simulink model "flex_robot_flat"  (R2020b)
settings: Solver=ode45  StartTime=0.0  StopTime=40  RelTol=1e-3
InitFcn:
  | params;
values from neighbouring files (symbols this model uses):
  param_controller = [c,d__1,d__2,m,g,l,I__1,I__2]    [params.m]
  param_system = [c,d__1,d__2,m,g,l,I__1,I__2]    [params.m]
  param_system_altered1 = [c*1.1,d__1,d__2,m,g,l,I__1,I__2]    [params.m]
  param_system_altered2 = [c*0.6,d__1,d__2,m,g,l,I__1,I__2]    [params.m]
  x__0 = [-pi/2,-pi/2,0,0]    [params.m]
undefined symbols (not defined in the file or in its folder): parReg
libraries: simulink_extras x6
settings Model: Creator=me  LastModifiedBy=simon
settings DataIOCC: LimitDataPoints=on  SaveFormat=Array  ReturnWorkspaceOutputs=off
settings OptimizationCC: BlockReduction=off  BooleanDataType=off  LifeSpan=inf
settings DebuggingCC: SaveWithParameterizedLinksMsg=none  UnderspecifiedInitializationDetection=Classic  MergeDetectMultiDrivingBlocksExec=none  SignalResolutionControl=TryResolveAllWithWarning  SFUnexpectedBacktrackingDiag=warning  SFNoUnconditionalDefaultTransitionDiag=warning  SFExecutionAtInitializationDiag=none  ArithmeticOperatorsInVariantConditions=warning
settings HardwareCC: ProdBitPerPointer=32  ProdBitPerSizeT=32  ProdBitPerPtrDiffT=32  ProdLargestAtomicFloat=None  ProdIntDivRoundTo=Undefined  ProdEndianess=Unspecified  ProdWordSize=32  ProdHWDeviceType=32-bit Generic  TargetUnknown=on
settings ModelReferenceCC: PropagateSignalLabelsOutOfModel=off
settings SFSimCC: SimUseLocalCustomCode=off  CustomCodeUndefinedFunction=UseInterfaceOnly
settings RTWCC: RTWUseLocalCustomCode=off
settings CodeAppCC: StateflowObjectComments=on
settings GRTTargetCC: TargetLangStandard=C89/C90 (ANSI)
settings ConfigComp: CovMetricSettings=dw  CovSaveCumulativeToWorkspaceVar=on  CovSaveSingleToWorkspaceVar=on  CovExternalEMLEnable=off

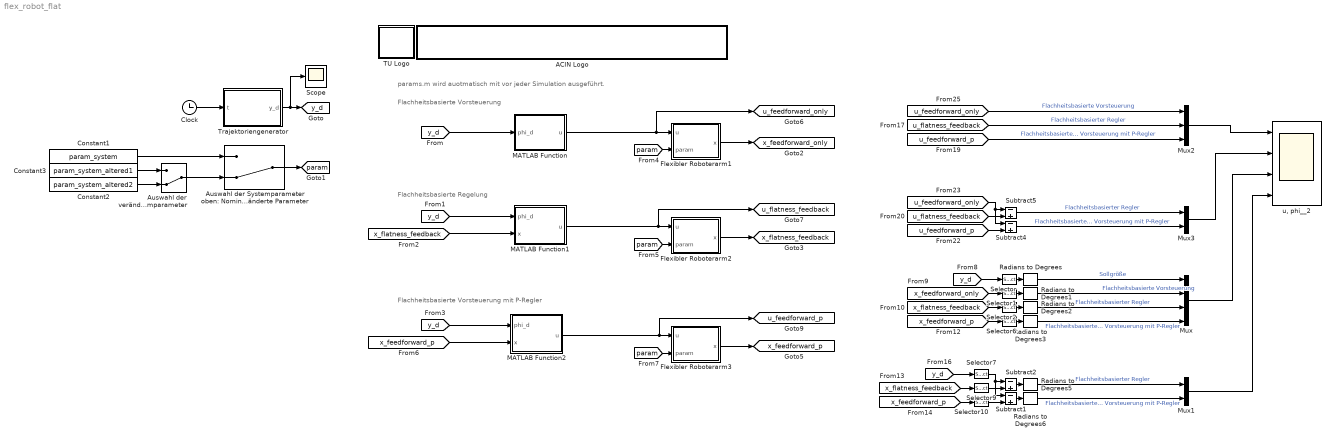
== system flex_robot_flat ==
  note: Flachheitsbasierte Vorsteuerung
  note: Flachheitsbasierte Regelung
  note: Flachheitsbasierte Vorsteuerung mit P-Regler
  note: params.m wird auotmatisch mit vor jeder Simulation ausgeführt.
  ACIN Logo : Subsystem
      mask init:
      | s = get_param(gcb,'UserData');
      mask Display:
      | image(s.logo,[0 0 439 45]);
      | %axis image
  Auswahl der veränderten Systemparameter : ManualSwitch  CurrentSetting=0
  Auswahl der Systemparameter oben: Nominelle Parameter unten: Veränderte Parameter : ManualSwitch  CurrentSetting=0
  Clock : Clock
  Constant1 : Constant  Value=param_system
  Constant2 : Constant  Value=param_system_altered2
  Constant3 : Constant  Value=param_system_altered1
  Flexibler Roboterarm1 : Subsystem
  Flexibler Roboterarm2 : Subsystem
  Flexibler Roboterarm3 : Subsystem
  MATLAB Function : MATLAB Function  TreatAsAtomicUnit=on
  MATLAB Function1 : MATLAB Function  TreatAsAtomicUnit=on
  MATLAB Function2 : MATLAB Function  TreatAsAtomicUnit=on
  Mux : Mux
  Mux1 : Mux  Inputs=2
  Mux2 : Mux  Inputs=3
  Mux3 : Mux  Inputs=2
  Radians to Degrees{,1..3,5..6} (6 alike) : simulink_extras/Transformations/Radians to Degrees
  Scope : Scope
  Selector : Selector  InputPortWidth=5  IndexOptions=Index vector (dialog)  Indices=[1]  OutputSizes=1
  Selector{1..2,6,9..10} (5 alike) : Selector  InputPortWidth=4  IndexOptions=Index vector (dialog)  Indices=2  OutputSizes=1
  Selector7 : Selector  InputPortWidth=5  IndexOptions=Index vector (dialog)  Indices=[1]  OutputSizes=1
  Subtract{1..2,4..5} (4 alike) : Sum  Inputs=-+
  TU Logo : Subsystem
      mask init:
      | s = get_param(gcb,'UserData');
      mask Display: image(s.logo,[0 0 45 45]);
  Trajektoriengenerator : MATLAB Function  TreatAsAtomicUnit=on
  "u, phi__2" : Scope  NumInputPorts=4
  tag scope: param=global, u_feedforward_only=global, u_feedforward_p=global, u_flatness_feedback=global, x_feedforward_only=global, x_feedforward_p=global, x_flatness_feedback=global, y_d=global
  wires:
  Clock/1 -> Trajektoriengenerator/1(t)
  Radians to Degrees/1 -> Mux/1  "Sollgröße"
  MATLAB Function1/1(u) -> [u_flatness_feedback], Flexibler Roboterarm2/1(u)
  Flexibler Roboterarm2/1(x) -> [x_flatness_feedback]
  Flexibler Roboterarm3/1(x) -> [x_feedforward_p]
  MATLAB Function2/1(u) -> [u_feedforward_p], Flexibler Roboterarm3/1(u)
  Constant1/1 -> Auswahl der Systemparameter oben: Nominelle Parameter unten: Veränderte Parameter/1
  Trajektoriengenerator/1(y_d) -> Scope/1, [y_d]
  [y_d] -> MATLAB Function/1(phi_d)
  [y_d] -> MATLAB Function1/1(phi_d)
  [y_d] -> MATLAB Function2/1(phi_d)
  Auswahl der Systemparameter oben: Nominelle Parameter unten: Veränderte Parameter/1 -> [param]
  [param] -> Flexibler Roboterarm1/2(param)
  [param] -> Flexibler Roboterarm2/2(param)
  [param] -> Flexibler Roboterarm3/2(param)
  Flexibler Roboterarm1/1(x) -> [x_feedforward_only]
  [y_d] -> Selector/1
  [x_feedforward_only] -> Selector1/1
  Radians to Degrees1/1 -> Mux/2  "Flachheitsbasierte Vorsteuerung"
  Radians to Degrees2/1 -> Mux/3  "Flachheitsbasierter Regler"
  [x_flatness_feedback] -> Selector2/1
  Radians to Degrees5/1 -> Mux1/1  "Flachheitsbasierter Regler"
  [x_feedforward_p] -> Selector10/1
  [x_flatness_feedback] -> Selector9/1
  Radians to Degrees6/1 -> Mux1/2  "Flachheitsbasierte Vorsteuerung mit P-Regler"
  Selector9/1 -> Subtract2/2
  Selector10/1 -> Subtract1/2
  Selector7/1 -> Subtract1/1, Subtract2/1
  [u_flatness_feedback] -> Mux2/2  "Flachheitsbasierter Regler"
  Subtract4/1 -> Mux3/2  "Flachheitsbasierte Vorsteuerung mit P-Regler"
  [u_flatness_feedback] -> Subtract5/2
  [u_feedforward_only] -> Subtract4/1, Subtract5/1
  Mux2/1 -> "u, phi__2"/1
  [u_feedforward_p] -> Subtract4/2
  Subtract5/1 -> Mux3/1  "Flachheitsbasierter Regler"
  [u_feedforward_only] -> Mux2/1  "Flachheitsbasierte Vorsteuerung"
  Mux3/1 -> "u, phi__2"/2
  Constant3/1 -> Auswahl der veränderten Systemparameter/1
  Constant2/1 -> Auswahl der veränderten Systemparameter/2
  Auswahl der veränderten Systemparameter/1 -> Auswahl der Systemparameter oben: Nominelle Parameter unten: Veränderte Parameter/2
  Radians to Degrees3/1 -> Mux/4  "Flachheitsbasierte Vorsteuerung mit P-Regler"
  [x_feedforward_p] -> Selector6/1
  [y_d] -> Selector7/1
  [u_feedforward_p] -> Mux2/3  "Flachheitsbasierte Vorsteuerung mit P-Regler"
  MATLAB Function/1(u) -> [u_feedforward_only], Flexibler Roboterarm1/1(u)
  Mux/1 -> "u, phi__2"/3
  Mux1/1 -> "u, phi__2"/4
  Selector/1 -> Radians to Degrees/1
  Selector1/1 -> Radians to Degrees1/1
  Selector2/1 -> Radians to Degrees2/1
  Selector6/1 -> Radians to Degrees3/1
  Subtract2/1 -> Radians to Degrees5/1
  Subtract1/1 -> Radians to Degrees6/1
  [x_flatness_feedback] -> MATLAB Function1/2(x)
  [x_feedforward_p] -> MATLAB Function2/2(x)

== system flex_robot_flat/ACIN Logo ==

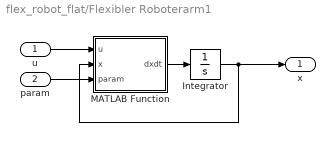
== system flex_robot_flat/Flexibler Roboterarm1 ==
  u : Inport
  param : Inport  Port=2
  Integrator : Integrator  InitialCondition=x__0
  MATLAB Function : MATLAB Function  TreatAsAtomicUnit=on
  x : Outport  VectorParamsAs1DForOutWhenUnconnected=off
  wires:
  u/1 -> MATLAB Function/1(u)
  Integrator/1 -> x/1, MATLAB Function/2(x)
  MATLAB Function/1(dxdt) -> Integrator/1
  param/1 -> MATLAB Function/3(param)

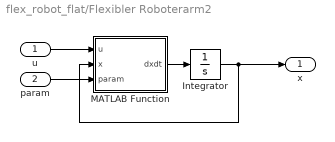
== system flex_robot_flat/Flexibler Roboterarm2 ==
  u : Inport
  param : Inport  Port=2
  Integrator : Integrator  InitialCondition=x__0
  MATLAB Function : MATLAB Function  TreatAsAtomicUnit=on
  x : Outport  VectorParamsAs1DForOutWhenUnconnected=off
  wires:
  u/1 -> MATLAB Function/1(u)
  Integrator/1 -> x/1, MATLAB Function/2(x)
  MATLAB Function/1(dxdt) -> Integrator/1
  param/1 -> MATLAB Function/3(param)

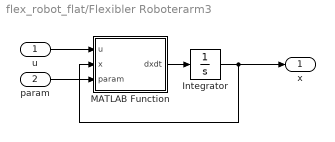
== system flex_robot_flat/Flexibler Roboterarm3 ==
  u : Inport
  param : Inport  Port=2
  Integrator : Integrator  InitialCondition=x__0
  MATLAB Function : MATLAB Function  TreatAsAtomicUnit=on
  x : Outport  VectorParamsAs1DForOutWhenUnconnected=off
  wires:
  u/1 -> MATLAB Function/1(u)
  Integrator/1 -> x/1, MATLAB Function/2(x)
  MATLAB Function/1(dxdt) -> Integrator/1
  param/1 -> MATLAB Function/3(param)

== system flex_robot_flat/TU Logo ==

== matlab function flex_robot_flat/MATLAB Function1 ==
  data: phi_d input; x input; u output; param_controller parameter; parReg parameter
function u = fcn(phi_d,x,param_controller,parReg)

% Sollwerte von phi2 und dessen Ableitungen
z__1 = phi_d(1);
z__2 = phi_d(2);
z__3 = phi_d(3);
z__4 = phi_d(4);
dz__4 = phi_d(5);

% Parameter des Systems
c = param_controller(1);
d__1 = param_controller(2);
d__2 = param_controller(3);
m = param_controller(4);
g = param_controller(5);
l = param_controller(6);
I__1 = param_controller(7);
I__2 = param_controller(8);

% Messgrößen
varphi__1 = x(1);
varphi__2 = x(2);
omega__1 = x(3);
omega__2 = x(4);

% Reglerparameter
a0 = parReg.a0;
a1 = parReg.a1;
a2 = parReg.a2;
a3 = parReg.a3;

% Stellgröße
u = 0.1e1 / c * I__2 * I__1 * (dz__4 + d__2 / I__2 ^ 2 * c * omega__1 - (m * g * l * cos(varphi__2) / I__2 * omega__2 - d__2 / I__2 ^ 2 * (-c + m * g * l * sin(varphi__2))) * omega__2 - c / I__2 * (-c * varphi__1 + c * varphi__2 - d__1 * omega__1) / I__1 - ((-c + m * g * l * sin(varphi__2)) / I__2 + d__2 ^ 2 / I__2 ^ 2) * (c * varphi__1 - c * varphi__2 - m * g * l * cos(varphi__2) - d__2 * omega__2) / I__2 - a0 * (-z__1 + varphi__2) - a1 * (-z__2 + omega__2) - a2 * ((c * varphi__1 - c * varphi__2 - m * g * l * cos(varphi__2) - d__2 * omega__2) / I__2 - z__3) - a3 * (c / I__2 * omega__1 + (-c + m * g * l * sin(varphi__2)) / I__2 * omega__2 - d__2 / I__2 ^ 2 * (c * varphi__1 - c * varphi__2 - m * g * l * cos(varphi__2) - d__2 * omega__2) - z__4));

== matlab function flex_robot_flat/MATLAB Function ==
  data: phi_d input; u output; param_controller parameter
function u = fcn(phi_d,param_controller)

% Sollwerte von phi2 und dessen Ableitungen
z__1 = phi_d(1);
z__2 = phi_d(2);
z__3 = phi_d(3);
z__4 = phi_d(4);
dz__4 = phi_d(5);

% Parameter des Systems
c = param_controller(1);
d__1 = param_controller(2);
d__2 = param_controller(3);
m = param_controller(4);
g = param_controller(5);
l = param_controller(6);
I__1 = param_controller(7);
I__2 = param_controller(8);

varphi__1 = (m * g * l * cos(z__1) + z__3 * I__2 + c * z__1 + d__2 * z__2) / c;
varphi__2 = z__1;
omega__1 = (-sin(z__1) * g * l * m * z__2 + I__2 * z__4 + c * z__2 + d__2 * z__3) / c;
omega__2 = z__2;

% Stellgröße
u = 0.1e1 / c * I__2 * I__1 * (d__2 / I__2 ^ 2 * c * omega__1 - (m * g * l * cos(varphi__2) / I__2 * omega__2 - d__2 / I__2 ^ 2 * (-c + m * g * l * sin(varphi__2))) * omega__2 - c / I__2 * (-c * varphi__1 + c * varphi__2 - d__1 * omega__1) / I__1 - ((-c + m * g * l * sin(varphi__2)) / I__2 + d__2 ^ 2 / I__2 ^ 2) * (c * varphi__1 - c * varphi__2 - m * g * l * cos(varphi__2) - d__2 * omega__2) / I__2 + dz__4);

== matlab function flex_robot_flat/MATLAB Function2 ==
  data: phi_d input; x input; u output; param_controller parameter; parReg parameter
function u = fcn(phi_d,x,param_controller,parReg)

% Sollwerte von phi2 und dessen Ableitungen
z__1 = phi_d(1);
z__2 = phi_d(2);
z__3 = phi_d(3);
z__4 = phi_d(4);
dz__4 = phi_d(5);

% Parameter des Systems
c = param_controller(1);
d__1 = param_controller(2);
d__2 = param_controller(3);
m = param_controller(4);
g = param_controller(5);
l = param_controller(6);
I__1 = param_controller(7);
I__2 = param_controller(8);

varphi__1 = (m * g * l * cos(z__1) + z__3 * I__2 + c * z__1 + d__2 * z__2) / c;
varphi__2 = z__1;
omega__1 = (-sin(z__1) * g * l * m * z__2 + I__2 * z__4 + c * z__2 + d__2 * z__3) / c;
omega__2 = z__2;

% Fehler
e = z__1-x(2);

% Stellgröße
u = 0.1e1 / c * I__2 * I__1 * (d__2 / I__2 ^ 2 * c * omega__1 - (m * g * l * cos(varphi__2) / I__2 * omega__2 - d__2 / I__2 ^ 2 * (-c + m * g * l * sin(varphi__2))) * omega__2 - c / I__2 * (-c * varphi__1 + c * varphi__2 - d__1 * omega__1) / I__1 - ((-c + m * g * l * sin(varphi__2)) / I__2 + d__2 ^ 2 / I__2 ^ 2) * (c * varphi__1 - c * varphi__2 - m * g * l * cos(varphi__2) - d__2 * omega__2) / I__2 + dz__4);
u = u + parReg.K*e;

== matlab function flex_robot_flat/Trajektoriengenerator ==
  data: t input; y_d output; param_trajectory parameter
function y_d  = trajgen(t,param_trajectory)
  T   = param_trajectory(1);
  a0 = param_trajectory(2);
  a1 = param_trajectory(3);

  % Generierung der Trajektorie y1d für den flachen Ausgang y1
  if (t<=0)
      phi__2_d     = a0;
      phi__2_dp    = 0;
      phi__2_dpp   = 0;
      phi__2_dppp  = 0;
      phi__2_dpppp = 0;
  elseif (t>T)
      phi__2_d     = a1;
      phi__2_dp    = 0;
      phi__2_dpp   = 0;
      phi__2_dppp  = 0;
      phi__2_dpppp = 0;
  else
      % Generierung der Solltrajektorie für q1
      phi__2_d     = a0 - 126 / T ^ 5 * (a0 - a1) * t ^ 5 + 420 / T ^ 6 * (a0 ...
          - a1) * t ^ 6 - 540 / T ^ 7 * (a0 - a1) * t ^ 7 + 315 / T ^ 8 * ...
          (a0 - a1) * t ^ 8 - 70 * (a0 - a1) / T ^ 9 * t ^ 9;
      % Generierung der ersten Ableitung der Solltrajektorie für q1
      phi__2_dp    = -630 / T ^ 5 * (a0 - a1) * t ^ 4 + 2520 / T ^ 6 * (a0 - ...
          a1) * t ^ 5 - 3780 / T ^ 7 * (a0 - a1) * t ^ 6 + 2520 / T ^ 8 * ...
          (a0 - a1) * t ^ 7 - 630 * (a0 - a1) / T ^ 9 * t ^ 8;
      % Generierung der zweiten Ableitung der Solltrajektorie für q1
      phi__2_dpp   =  -2520 / T ^ 5 * (a0 - a1) * t ^ 3 + 12600 / T ^ 6 * (a0 - ...
          a1) * t ^ 4 - 22680 / T ^ 7 * (a0 - a1) * t ^ 5 + 17640 / T ^ 8 * ...
          (a0 - a1) * t ^ 6 - 5040 * (a0 - a1) / T ^ 9 * t ^ 7;
      % Generierung der dritten Ableitung der Solltrajektorie für q1
      phi__2_dppp  = -7560 / T ^ 5 * (a0 - a1) * t ^ 2 + 50400 / T ^ 6 * (a0 - ...
          a1) * t ^ 3 - 113400 / T ^ 7 * (a0 - a1) * t ^ 4 + 105840 / T ^ 8 ...
          * (a0 - a1) * t ^ 5 - 35280 * (a0 - a1) / T ^ 9 * t ^ 6;
      % Generierung der vierten Ableitung der Solltrajektorie für q1
      phi__2_dpppp =  -15120 / T ^ 5 * (a0 - a1) * t + 151200 / T ^ 6 * (a0 - ...
          a1) * t ^ 2 - 453600 / T ^ 7 * (a0 - a1) * t ^ 3 + 529200 / T ^ 8 ...
          * (a0 - a1) * t ^ 4 - 211680 * (a0 - a1) / T ^ 9 * t ^ 5;
  end
  % Verpacken der Solltrajektorie samt Ableitungen in einem Vektor zur Uebergabe
  % an die Vorsteuerung
  y_d = [phi__2_d,phi__2_dp,phi__2_dpp,phi__2_dppp,phi__2_dpppp];
end

== matlab function flex_robot_flat/Flexibler Roboterarm2/MATLAB Function ==
  data: u input; dxdt output; x input; param input
function dxdt = fcn(u,x,param)
  c=param(1);
  d__1=param(2);
  d__2=param(3);
  m=param(4);
  g=param(5);
  l=param(6);
  I__1=param(7);
  I__2=param(8);
  
  varphi__1=x(1);
  varphi__2=x(2);
  omega__1=x(3);
  omega__2=x(4);
  
  dxdt=zeros(4,1);
  dxdt(1) = omega__1;
  dxdt(2) = omega__2;
  dxdt(3) = -c/I__1*varphi__1 + c/I__1*varphi__2 - d__1/I__1*omega__1 + 1/I__1*u;
  dxdt(4) =  c/I__2*varphi__1 - c/I__2*varphi__2 - m*g*l/I__2*cos(varphi__2) - d__2/I__2*omega__2;
end

== matlab function flex_robot_flat/Flexibler Roboterarm3/MATLAB Function ==
  data: u input; dxdt output; x input; param input
function dxdt = fcn(u,x,param)
  c=param(1);
  d__1=param(2);
  d__2=param(3);
  m=param(4);
  g=param(5);
  l=param(6);
  I__1=param(7);
  I__2=param(8);
  
  varphi__1=x(1);
  varphi__2=x(2);
  omega__1=x(3);
  omega__2=x(4);
  
  dxdt=zeros(4,1);
  dxdt(1) = omega__1;
  dxdt(2) = omega__2;
  dxdt(3) = -c/I__1*varphi__1 + c/I__1*varphi__2 - d__1/I__1*omega__1 + 1/I__1*u;
  dxdt(4) =  c/I__2*varphi__1 - c/I__2*varphi__2 - m*g*l/I__2*cos(varphi__2) - d__2/I__2*omega__2;
end

== matlab function flex_robot_flat/Flexibler Roboterarm1/MATLAB Function ==
  data: u input; dxdt output; x input; param input
function dxdt = fcn(u,x,param)
  c=param(1);
  d__1=param(2);
  d__2=param(3);
  m=param(4);
  g=param(5);
  l=param(6);
  I__1=param(7);
  I__2=param(8);
  
  varphi__1=x(1);
  varphi__2=x(2);
  omega__1=x(3);
  omega__2=x(4);
  
  dxdt=zeros(4,1);
  dxdt(1) = omega__1;
  dxdt(2) = omega__2;
  dxdt(3) = -c/I__1*varphi__1 + c/I__1*varphi__2 - d__1/I__1*omega__1 + 1/I__1*u;
  dxdt(4) =  c/I__2*varphi__1 - c/I__2*varphi__2 - m*g*l/I__2*cos(varphi__2) - d__2/I__2*omega__2;
end
